simulink model "kaffeeautomat_2"  (R2015b)
settings: Solver=FixedStepAuto  StartTime=0.0  StopTime=60  RelTol=1e-3
libraries: simulink x1
settings Model: Creator=scco1019  LastModifiedBy=scco1019

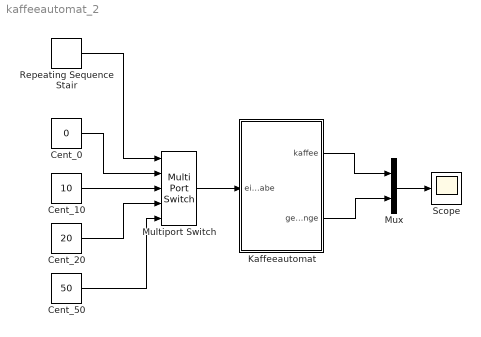
== system kaffeeautomat_2 ==
  Cent_0 : Constant  Value=0
  Cent_10 : Constant  Value=10
  Cent_20 : Constant  Value=20
  Cent_50 : Constant  Value=50
  Kaffeeautomat : Stateflow chart  TreatAsAtomicUnit=on
  Multiport Switch : MultiPortSwitch  Inputs=4
  Mux : Mux  Inputs=2
  Repeating Sequence Stair : simulink/Sources/Repeating Sequence Stair  OutValues=[1 2 2 2 2 2 1 2 3 3 1 4 1 2 2 3 3 1 2 2 1 1 1 1 4 1].'  tsamp=-1  OutMin=[]  OutMax=[]  OutDataTypeStr=double  OutputDataTypeScalingMode=double  OutDataType=fixdt(0,8)  ConRadixGroup=Best Precision: Vector-wise  OutScaling=2^-12
  Scope : Scope
  wires:
  Multiport Switch/1 -> Kaffeeautomat/1(eingabe)
  Repeating Sequence Stair/1 -> Multiport Switch/1
  Cent_0/1 -> Multiport Switch/2
  Cent_10/1 -> Multiport Switch/3
  Cent_20/1 -> Multiport Switch/4
  Cent_50/1 -> Multiport Switch/5
  Kaffeeautomat/2(geldmenge) -> Mux/2
  Kaffeeautomat/1(kaffee) -> Mux/1
  Mux/1 -> Scope/1

== stateflow chart kaffeeautomat_2/Kaffeeautomat ==
  state Kein_Kaffee/
  state Kaffee/
    entry: kaffee=1
  (default) -> Kein_Kaffee : {geldmenge=0}
  Kein_Kaffee -> Kein_Kaffee [order 1] : [eingabe==10]
      | {geldmenge=geldmenge+10}
  Kein_Kaffee -> Kein_Kaffee [order 4] : [eingabe==20]
      | {geldmenge=geldmenge+20}
  Kein_Kaffee -> Kein_Kaffee [order 3] : [eingabe==50]
      | {geldmenge=geldmenge+50}
  Kaffee -> Kein_Kaffee : {geldmenge=geldmenge-50;
      | kaffee=0}
  Kein_Kaffee -> Kaffee [order 2] : [geldmenge>=50]
  data: eingabe input; kaffee output; geldmenge output
